simulink model "HVDCMMCInterconnection"  (R2023b)
settings: Solver=FixedStepDiscrete  StartTime=0.0  StopTime=10  FixedStep=Ts_Power  RelTol=1e-4
PreLoadFcn:
  | HVDCMMCInterconnectionParam
StartFcn:
  | tic
StopFcn:
  | toc
values from neighbouring files (symbols this model uses):
  C_PM = 1.758e-3    (= 0.001758)    [HVDCMMCInterconnectionParam.m]
  Cg = 50e-9    (= 5e-08)    [HVDCMMCInterconnectionParam.m]
  D_R = 0.001    [HVDCMMCInterconnectionParam.m]
  D_Rs = 1e8    (= 100000000)    [HVDCMMCInterconnectionParam.m]
  D_Vf = 0    [HVDCMMCInterconnectionParam.m]
  Fnom = 50    [HVDCMMCInterconnectionParam.m]
  HRM = 2    [HVDCMMCInterconnectionParam.m]
  Ki_Ireg = 6    [HVDCMMCInterconnectionParam.m]
  Ki_Preg = 1.0    (= 1)    [HVDCMMCInterconnectionParam.m]
  Ki_Qreg = 1.0    (= 1)    [HVDCMMCInterconnectionParam.m]
  Ki_VDCreg = 100    [HVDCMMCInterconnectionParam.m]
  Kp_Ireg = 0.6    [HVDCMMCInterconnectionParam.m]
  Kp_Preg = 0.5/3    (= 0.166666666667)    [HVDCMMCInterconnectionParam.m]
  Kp_Qreg = 0.5/3    (= 0.166666666667)    [HVDCMMCInterconnectionParam.m]
  Kp_VDCreg = 4    [HVDCMMCInterconnectionParam.m]
  L_cable = 15e-3    (= 0.015)    [HVDCMMCInterconnectionParam.m]
  Larm = Larm_pu*(Zb_ac/(2*pi*Fnom))    [HVDCMMCInterconnectionParam.m]
  Lff = Larm_pu/2    (= 0.075)    [HVDCMMCInterconnectionParam.m]
  Limits_Ireg = [ 2.0  -2.0]    [HVDCMMCInterconnectionParam.m]
  Limits_Preg = [ 1.2, 0.8 ]    [HVDCMMCInterconnectionParam.m]
  Limits_Qreg = [ 0.25, -0.25 ]    [HVDCMMCInterconnectionParam.m]
  Limits_VDCreg = [ 2.0  -2.0]    [HVDCMMCInterconnectionParam.m]
  Lxfo = 0.12    [HVDCMMCInterconnectionParam.m]
  Nb_PM = 36    [HVDCMMCInterconnectionParam.m]
  Pnom = 1000e6    (= 1000000000)    [HVDCMMCInterconnectionParam.m]
  R_cable = 0.5    [HVDCMMCInterconnectionParam.m]
  R_startup = 400    [HVDCMMCInterconnectionParam.m]
  Rarm = Rarm_pu*Zb_ac    [HVDCMMCInterconnectionParam.m]
  Rff = Rarm_pu/2    (= 0.00075)    [HVDCMMCInterconnectionParam.m]
  Rg = 100    [HVDCMMCInterconnectionParam.m]
  Rxfo = 0.003    [HVDCMMCInterconnectionParam.m]
  Slope_Pref = 0.5    [HVDCMMCInterconnectionParam.m]
  Slope_Qref = 0.5    [HVDCMMCInterconnectionParam.m]
  Slope_Vdc_ref = Vnom_dc/5    (= 128000)    [HVDCMMCInterconnectionParam.m]
  Tbrk1_On = 0.1    [HVDCMMCInterconnectionParam.m]
  Tbrk2_On = 1.0    (= 1)    [HVDCMMCInterconnectionParam.m]
  Tdeblock = 1.5    [HVDCMMCInterconnectionParam.m]
  Tfault = 9999    [HVDCMMCInterconnectionParam.m]
  Ton_Converter2 = 4    [HVDCMMCInterconnectionParam.m]
  Ton_PQreg = 4    [HVDCMMCInterconnectionParam.m]
  Ton_VDCreg = 1.5    [HVDCMMCInterconnectionParam.m]
  Ts = Ts_Control    (= 4e-05)    [HVDCMMCInterconnectionParam.m]    (also in power_circ2ss_sps_calc.m = 1e-06)
  Ts_Control = 40e-6    (= 4e-05)    [HVDCMMCInterconnectionParam.m]
  Ts_Power = 20e-6    (= 2e-05)    [HVDCMMCInterconnectionParam.m]
  Vb_ac = sqrt(2/3)*Vnom_sec    [HVDCMMCInterconnectionParam.m]
  Vb_dc = Vnom_dc    (= 640000)    [HVDCMMCInterconnectionParam.m]
  Vc0_PM = 0    [HVDCMMCInterconnectionParam.m]
  Vnom_dc = 640e3    (= 640000)    [HVDCMMCInterconnectionParam.m]
  Vnom_prim = 400e3    (= 400000)    [HVDCMMCInterconnectionParam.m]
  Vnom_sec = 333e3    (= 333000)    [HVDCMMCInterconnectionParam.m]
  w = 2*pi*Fnom    (= 314.159265359)    [HVDCMMCInterconnectionParam.m]
undefined symbols (not defined in the file or in its folder): ACDC, ACDC3, DiscIntNeverNeededParam, gcbh, Pcc, S, sps_AC, sps_rtmsupport
libraries: simulink x61, spsControlledVoltageSourceLib x56, spsCurrentMeasurementLib x56, spsDiodeLib x40, spsSeriesRLCBranchLib x32, spsVoltageMeasurementLib x20, powerlib_extras x9, spsHalfBridgeMMCmodel x8, spsGroundLib x7, spsSecondOrderFilterLib x6, spsabctodq0Lib x6, spsMeanLib x3
(part 8 of 11)

== system HVDCMMCInterconnection/MMC/An ==
  Uref : Inport
  Add1 : Sum  Commented=on  Inputs=+-
  Add2 : Sum  Commented=on  Inputs=-+
  An_Db : spsDiodeLib/Diode  Ron=D_R  Lon=0  Vf=D_Vf  IC=0  UseSnubber=0  Rs=D_Rs  Cs=D_Cs  Measurements=on
  An_Dt : spsDiodeLib/Diode  Ron=D_R  Lon=0  Vf=D_Vf  IC=0  UseSnubber=0  Rs=D_Rs  Cs=D_Cs  Measurements=on
  An_Icap : spsCurrentMeasurementLib/Current Measurement  PhasorSimulation=off  OutputType=Complex  PSBequivalent=0
  An_Ipos : spsCurrentMeasurementLib/Current Measurement  PhasorSimulation=off  OutputType=Complex  PSBequivalent=0
  An_Vbl : spsControlledVoltageSourceLib/Controlled Voltage Source  Initialize=on  Source_Type=AC  Amplitude=0  Phase=0  Frequency=0  Measurements=None
  An_Vin : spsControlledVoltageSourceLib/Controlled Voltage Source  Initialize=on  Source_Type=AC  Amplitude=0  Phase=0  Frequency=0  Measurements=None
  Bus Selector1 : BusSelector  OutputSignals=Diode current
  Bus Selector2 : BusSelector  OutputSignals=Diode current
  Compare To Constant1 : simulink/Logic and Bit Operations/Compare To Constant  Commented=on  relop=<=  const=0.5  OutDataTypeStr=boolean
  Constant3 : Constant  Commented=on  Value=ones(1,1)
  Constant4 : Constant  Commented=on  Value=ones(1,1)
  Data Type Conversion2 : DataTypeConversion  Commented=on  OutDataTypeStr=double  SaturateOnIntegerOverflow=off  RndMeth=Floor
  Demux : Demux  Outputs=2
  Demux2 : Demux  Outputs=2
  Demux5 : Demux  Outputs=2
  Discrete-Time Integrator1 : DiscreteIntegrator  IntegratorMethod=Integration: Trapezoidal  gainval=1  InitialCondition=Vc_Initial  SampleTime=Ts  UpperSaturationLimit=5000  LowerSaturationLimit=500  ICPrevOutput=DiscIntNeverNeededParam  ICPrevScaledInput=DiscIntNeverNeededParam
  From11 : From  Commented=on  GotoTag=uref
  From13 : From  Commented=on  GotoTag=Blk  TagVisibility=global
  Gain1 : Gain  Gain=n
  Gain4 : Gain  Gain=1/(C*n)
  Gain5 : Gain  Gain=2
  Mux1 : Mux  Inputs=2
  Mux2 : Mux  Inputs=2
  Mux3 : Mux  Commented=on  Inputs=2
  Mux7 : Mux  Inputs=2
  Product1 : Product  Commented=on
  Product3 : Product
  Product4 : Product
  Product5 : Product  Commented=on
  Product7 : Product
  Saturation : Saturate  Commented=on  UpperLimit=1  LowerLimit=-1
  Scope : Scope  Commented=on  NumInputPorts=2
  Sum3 : Sum  Inputs=1  InputSameDT=on  SaturateOnIntegerOverflow=on  OutDataTypeStr=Inherit: Same as first input
  Sum4 : Sum  Inputs=+-  InputSameDT=on  SaturateOnIntegerOverflow=on  OutDataTypeStr=Inherit: Same as first input
  Unit Delay5 : UnitDelay  InitialCondition=Vc_Initial  SampleTime=Ts  HasFrameUpgradeWarning=on
  Unit Delay6 : UnitDelay  InitialCondition=Vc_Initial  SampleTime=Ts  HasFrameUpgradeWarning=on
  Unit Delay7 : UnitDelay  SampleTime=Ts  HasFrameUpgradeWarning=on
  An_pos : PMIOPort  Side=Left
  An_neg : PMIOPort  Port=2  Side=Left
  Vc : Outport  VectorParamsAs1DForOutWhenUnconnected=off
  tag scope: An_Vbl_EMT=global, An_Vin_EMT=global, I_An_Db_EMT=global, I_An_Dt_EMT=global
  wires:
  Demux/1 -> [An_Vin_EMT]
  [An_Vin_EMT] -> An_Vin/1
  Product3/1 -> Sum3/1
  Demux/2 -> [An_Vbl_EMT]
  [Ipos] -> Mux1/1
  Unit Delay5/1 -> Sum4/2
  Gain5/1 -> Sum4/1
  Sum4/1 -> Product7/2, Product4/2, Vc/1  "Vc"
  Discrete-Time Integrator1/1 -> Unit Delay6/1
  Mux2/1 -> Demux/1
  [An_Vbl_EMT] -> An_Vbl/1
  [Icap] -> Mux1/2
  Gain4/1 -> Discrete-Time Integrator1/1
  Unit Delay6/1 -> Gain5/1, Unit Delay5/1
  Mux1/1 -> Unit Delay7/1
  Mux7/1 -> Gain1/1
  Demux2/1 -> Product4/1
  Demux2/2 -> Product7/1
  Product4/1 -> Mux2/1  "Vin"
  Product7/1 -> Mux2/2  "Vbl"
  Demux5/2 -> [ublk]
  [uref] -> Mux7/1
  [ublk] -> Mux7/2
  An_Ipos/1 -> [Ipos]
  An_Icap/1 -> [Icap]
  Unit Delay7/1 -> Product3/2
  Gain1/1 -> Demux2/1, Product3/1
  Demux5/1 -> [uref]
  Uref/1 -> Demux5/1
  Data Type Conversion2/1 -> Product5/1, Product1/1
  From13/1 -> Compare To Constant1/1
  Add2/1 -> Add1/2, Product5/2
  Constant4/1 -> Add1/1
  From11/1 -> Saturation/1
  Compare To Constant1/1 -> Data Type Conversion2/1
  Add1/1 -> Product1/2
  Product1/1 -> Mux3/1
  Constant3/1 -> Add2/2
  Saturation/1 -> Add2/1
  Sum3/1 -> Gain4/1
  Product5/1 -> Mux3/2
  Bus Selector2/1 -> [I_An_Dt_EMT]  "<Diode current>"
  An_Dt/1 -> Bus Selector2/1
  Bus Selector1/1 -> [I_An_Db_EMT]  "<Diode current>"
  An_Db/1 -> Bus Selector1/1
  connections:
  An_Ipos/RConn1 -- An_Dt/LConn1 -- An_Db/RConn1
  An_Vbl/LConn1 -- An_neg/RConn1 -- An_Db/LConn1
  An_Vbl/RConn1 -- An_Icap/RConn1
  An_Dt/RConn1 -- An_Icap/LConn1
  An_pos/RConn1 -- An_Vin/RConn1
  An_Vin/LConn1 -- An_Ipos/LConn1

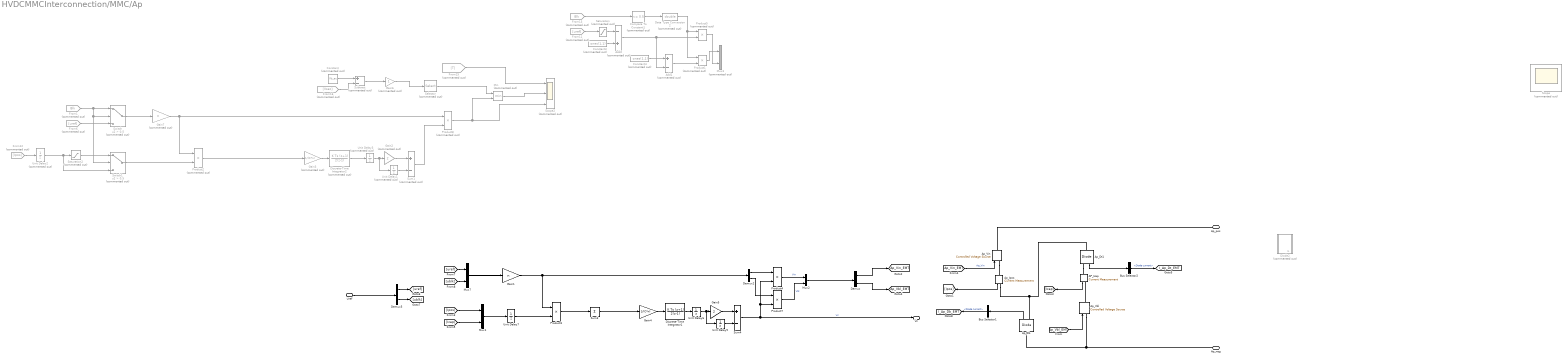
== system HVDCMMCInterconnection/MMC/Ap ==
  Uref : Inport
  AP_Icap : spsCurrentMeasurementLib/Current Measurement  PhasorSimulation=off  OutputType=Complex  PSBequivalent=0
  Add1 : Sum  Commented=on  Inputs=+-
  Add2 : Sum  Commented=on  Inputs=-+
  Ap_Db : spsDiodeLib/Diode  Ron=D_R  Lon=0  Vf=D_Vf  IC=0  UseSnubber=0  Rs=D_Rs  Cs=D_Cs  Measurements=on
  Ap_Dt1 : spsDiodeLib/Diode  Ron=D_R  Lon=0  Vf=D_Vf  IC=0  UseSnubber=0  Rs=D_Rs  Cs=D_Cs  Measurements=on
  Ap_Ipos : spsCurrentMeasurementLib/Current Measurement  PhasorSimulation=off  OutputType=Complex  PSBequivalent=0
  Ap_Vbl : spsControlledVoltageSourceLib/Controlled Voltage Source  Initialize=on  Source_Type=AC  Amplitude=0  Phase=0  Frequency=0  Measurements=None
  Ap_Vin : spsControlledVoltageSourceLib/Controlled Voltage Source  Initialize=on  Source_Type=AC  Amplitude=0  Phase=0  Frequency=0  Measurements=None
  Bus Selector1 : BusSelector  OutputSignals=Diode current
  Bus Selector2 : BusSelector  OutputSignals=Diode current
  Compare To Constant1 : simulink/Logic and Bit Operations/Compare To Constant  Commented=on  relop=<=  const=0.5  OutDataTypeStr=boolean
  Constant : Constant  Commented=on  Value=Vb_ac
  Constant3 : Constant  Commented=on  Value=ones(1,1)
  Constant4 : Constant  Commented=on  Value=ones(1,1)
  Data Type Conversion2 : DataTypeConversion  Commented=on  OutDataTypeStr=double  SaturateOnIntegerOverflow=off  RndMeth=Floor
  Demux : Demux  Outputs=2
  Demux2 : Demux  Outputs=2
  Demux5 : Demux  Outputs=2
  Diode2 : Subsystem  Commented=on  AncestorBlock=sps_lib/Power Electronics/Diode2  DialogController=POWERSYS.PowerSysDialog  LoadFcn=sps_rtmsupport('LoadFcn',gcbh);  StartFcn=sps_rtmsupport('StartFcn',gcbh);  StopFcn=sps_rtmsupport('StopFcn',gcbh);  mask(Diode){Ron=D_R, Lon=0, Vf=D_Vf, IC=0, UseSnubber=0, Rs=D_Rs, Cs=inf, Measurements=on}
      mask prompts: Ron "Resistance Ron (Ohms) :"; Lon "Inductance Lon (H) :"; Vf "Forward voltage Vf (V) :"; IC "Initial current Ic (A) :"; UseSnubber "Snubber"; Rs "Snubber resistance Rs (Ohms) :"; Cs "Snubber capacitance Cs (F) :"; Measurements "Show measurement port"
      mask help:
      | Implements a diode in parallel with a series RC snubber circuit.
      | In on-state the Diode model has an internal resistance (Ron) and inductance (Lon).
      | For most applications the internal inductance should be set to zero.
      | The Diode impedance is infinite in off-state mode.
      mask init:
      | block = gcb;
      | [WantBlockChoice,Ts,X,Y,Ron,Vf] = powericon('SwitchesInit','Diode',block,Rs,Cs,Ron,Vf);
      | powericon('SetInternalModels','set',block,WantBlockChoice);
      settings: LibrarySourceBlock=sps_lib/Power Electronics/Diode2  CopyFcn=sps_rtmsupport('CopyFcn',gcbh); powericon('SwitchesCopyFcn','Diode',gcb)  DeleteFcn=sps_rtmsupport('DeleteFcn',gcbh);  UndoDeleteFcn=sps_rtmsupport('UndoDeleteFcn',gcbh);  ModelCloseFcn=sps_rtmsupport('ModelCloseFcn',gcbh);  PreSaveFcn=sps_rtmsupport('PreSaveFcn',gcbh);  PostSaveFcn=sps_rtmsupport('PostSaveFcn',gcbh);  NameChangeFcn=sps_rtmsupport('NameChangeFcn',gcbh);  PreCopyFcn=sps_rtmsupport('PreCopyFcn',gcbh);  OpenFcn=sps_rtmsupport('OpenFcn',gcbh, [5 8]);  CloseFcn=sps_rtmsupport('CloseFcn',gcbh);  PreDeleteFcn=sps_rtmsupport('PreDeleteFcn',gcbh);
      mask Help: helpview(psbhelp);
      mask Callback Ron: powericon('SwitchesEnables',gcb,'Diode');
      mask Callback Measurements:
      | powericon('OutputMCback',gcb);
      | %sps_rtmsupport('parametereditingmodes',gcbh, [5 8]);
      mask Display: plot(X.p1,Y.p1,X.p2,Y.p2,X.p3,Y.p3,X.p4,Y.p4,X.p5,Y.p5,X.p6,Y.p6)
  Discrete-Time Integrator1 : DiscreteIntegrator  IntegratorMethod=Integration: Trapezoidal  gainval=1  InitialCondition=Vc_Initial  SampleTime=Ts  UpperSaturationLimit=5000  LowerSaturationLimit=500  ICPrevOutput=DiscIntNeverNeededParam  ICPrevScaledInput=DiscIntNeverNeededParam
  Discrete-Time Integrator2 : DiscreteIntegrator  Commented=on  IntegratorMethod=Integration: Trapezoidal  gainval=1  InitialCondition=Vc_Initial  SampleTime=Ts  UpperSaturationLimit=5000  LowerSaturationLimit=500  ICPrevOutput=DiscIntNeverNeededParam  ICPrevScaledInput=DiscIntNeverNeededParam
  From1 : From  Commented=on  GotoTag=Blk  TagVisibility=global
  From11 : From  Commented=on  GotoTag=uref
  From12 : From  Commented=on  GotoTag=Ipos
  From13 : From  Commented=on  GotoTag=Blk  TagVisibility=global
  From15 : From  Commented=on  GotoTag=T
  From16 : From  Commented=on  GotoTag=Vsec  TagVisibility=global
  From6 : From  Commented=on  GotoTag=uref
  Gain1 : Gain  Gain=n
  Gain2 : Gain  Commented=on  Gain=2
  Gain3 : Gain  Commented=on  Gain=1/(C*n)
  Gain4 : Gain  Gain=1/(C*n)
  Gain5 : Gain  Gain=2
  Gain6 : Gain  Commented=on
  Gain7 : Gain  Commented=on  Gain=n
  Min : MinMax  Commented=on  Inputs=2
  Mux1 : Mux  Inputs=2
  Mux2 : Mux  Inputs=2
  Mux3 : Mux  Commented=on  Inputs=2
  Mux7 : Mux  Inputs=2
  Product{1..2,5,8} (4 alike) : Product  Commented=on
  Product3 : Product
  Product4 : Product
  Product7 : Product
  Saturation : Saturate  Commented=on  UpperLimit=1  LowerLimit=-1
  Saturation2 : Saturate  Commented=on  UpperLimit=inf  LowerLimit=0
  Scope : Scope  Commented=on  NumInputPorts=2
  Scope2 : Scope  Commented=on  NumInputPorts=3
  Selector : Selector  Commented=on  InputPortWidth=3  IndexOptions=Index vector (dialog)  Indices=[1]  OutputSizes=1
  Subtract : Sum  Commented=on  Inputs=+-
  Sum1 : Sum  Commented=on  Inputs=+-  InputSameDT=on  SaturateOnIntegerOverflow=on  OutDataTypeStr=Inherit: Same as first input
  Sum3 : Sum  Inputs=1  InputSameDT=on  SaturateOnIntegerOverflow=on  OutDataTypeStr=Inherit: Same as first input
  Sum4 : Sum  Inputs=+-  InputSameDT=on  SaturateOnIntegerOverflow=on  OutDataTypeStr=Inherit: Same as first input
  Switch : Switch  Commented=on  Criteria=u2 > Threshold  Threshold=0.5  SaturateOnIntegerOverflow=off  InputSameDT=off
  Switch1 : Switch  Commented=on  Criteria=u2 > Threshold  Threshold=0.5  SaturateOnIntegerOverflow=off  InputSameDT=off
  Unit Delay1 : UnitDelay  Commented=on  InitialCondition=Vc_Initial  SampleTime=Ts  HasFrameUpgradeWarning=on
  Unit Delay2 : UnitDelay  Commented=on  SampleTime=Ts  HasFrameUpgradeWarning=on
  Unit Delay3 : UnitDelay  Commented=on  InitialCondition=Vc_Initial  SampleTime=Ts  HasFrameUpgradeWarning=on
  Unit Delay5 : UnitDelay  InitialCondition=Vc_Initial  SampleTime=Ts  HasFrameUpgradeWarning=on
  Unit Delay6 : UnitDelay  InitialCondition=Vc_Initial  SampleTime=Ts  HasFrameUpgradeWarning=on
  Unit Delay7 : UnitDelay  SampleTime=Ts  HasFrameUpgradeWarning=on
  Ap_pos : PMIOPort  Side=Left
  Ap_neg : PMIOPort  Port=2  Side=Left
  Vc : Outport  VectorParamsAs1DForOutWhenUnconnected=off
  tag scope: Ap_Vbl_EMT=global, Ap_Vin_EMT=global, I_Ap_Db_EMT=global, I_Ap_Dt_EMT=global
  wires:
  Demux/1 -> [Ap_Vin_EMT]
  [Ap_Vin_EMT] -> Ap_Vin/1  "Ap_Vin"
  Product3/1 -> Sum3/1
  Demux/2 -> [Ap_Vbl_EMT]
  [Ipos] -> Mux1/1
  Unit Delay5/1 -> Sum4/2
  Gain5/1 -> Sum4/1
  Sum4/1 -> Product7/2, Product4/2, Vc/1  "Vc"
  Discrete-Time Integrator1/1 -> Unit Delay6/1
  Mux2/1 -> Demux/1
  [Ap_Vbl_EMT] -> Ap_Vbl/1
  [Icap] -> Mux1/2
  Gain4/1 -> Discrete-Time Integrator1/1
  Unit Delay6/1 -> Gain5/1, Unit Delay5/1
  Mux1/1 -> Unit Delay7/1
  Mux7/1 -> Gain1/1
  Demux2/1 -> Product4/1
  Demux2/2 -> Product7/1
  Product4/1 -> Mux2/1  "Vin"
  Product7/1 -> Mux2/2  "Vbl"
  Demux5/2 -> [ublk]
  [uref] -> Mux7/1
  [ublk] -> Mux7/2
  Ap_Ipos/1 -> [Ipos]
  AP_Icap/1 -> [Icap]
  Unit Delay7/1 -> Product3/2
  Gain1/1 -> Demux2/1, Product3/1
  Demux5/1 -> [uref]
  Uref/1 -> Demux5/1
  Data Type Conversion2/1 -> Product5/1, Product1/1
  From13/1 -> Compare To Constant1/1
  Add2/1 -> Add1/2, Product5/2
  Constant4/1 -> Add1/1
  From11/1 -> Saturation/1
  Compare To Constant1/1 -> Data Type Conversion2/1
  Add1/1 -> Product1/2
  Product1/1 -> Mux3/1
  Constant3/1 -> Add2/2
  Saturation/1 -> Add2/1
  Sum3/1 -> Gain4/1
  Product5/1 -> Mux3/2
  From1/1 -> Switch1/2, Switch/2, Switch/1
  Saturation2/1 -> Switch1/1
  Gain7/1 -> Product2/1, Product8/1
  Unit Delay3/1 -> Gain2/1, Unit Delay1/1
  Sum1/1 -> Product8/2
  Switch/1 -> Gain7/1
  Switch1/1 -> Product2/2
  From6/1 -> Switch/3
  Unit Delay2/1 -> Saturation2/1, Switch1/3
  Gain3/1 -> Discrete-Time Integrator2/1
  Discrete-Time Integrator2/1 -> Unit Delay3/1
  Unit Delay1/1 -> Sum1/2
  From12/1 -> Unit Delay2/1
  Product2/1 -> Gain3/1
  Gain2/1 -> Sum1/1
  Product8/1 -> Min/2, Scope2/3
  From16/1 -> Subtract/2
  Constant/1 -> Subtract/1
  Subtract/1 -> Gain6/1
  Gain6/1 -> Selector/1
  Selector/1 -> Min/1
  Min/1 -> Scope2/2
  From15/1 -> Scope2/1
  Bus Selector1/1 -> [I_Ap_Db_EMT]  "<Diode current>"
  Ap_Db/1 -> Bus Selector1/1
  Ap_Dt1/1 -> Bus Selector2/1
  Bus Selector2/1 -> [I_Ap_Dt_EMT]  "<Diode current>"
  connections:
  Ap_Ipos/RConn1 -- Ap_Dt1/LConn1 -- Ap_Db/RConn1
  Ap_Vbl/LConn1 -- Ap_neg/RConn1 -- Ap_Db/LConn1
  Ap_Vbl/RConn1 -- AP_Icap/RConn1
  Ap_Dt1/RConn1 -- AP_Icap/LConn1
  Ap_pos/RConn1 -- Ap_Vin/RConn1
  Ap_Vin/LConn1 -- Ap_Ipos/LConn1

== system HVDCMMCInterconnection/MMC/Bn ==
  Uref : Inport
  Bn_Db : spsDiodeLib/Diode  Ron=D_R  Lon=0  Vf=D_Vf  IC=0  UseSnubber=0  Rs=D_Rs  Cs=D_Cs  Measurements=on
  Bn_Dt : spsDiodeLib/Diode  Ron=D_R  Lon=0  Vf=D_Vf  IC=0  UseSnubber=0  Rs=D_Rs  Cs=D_Cs  Measurements=on
  Bn_Icap : spsCurrentMeasurementLib/Current Measurement  PhasorSimulation=off  OutputType=Complex  PSBequivalent=0
  Bn_Ipos : spsCurrentMeasurementLib/Current Measurement  PhasorSimulation=off  OutputType=Complex  PSBequivalent=0
  Bn_Vbl : spsControlledVoltageSourceLib/Controlled Voltage Source  Initialize=on  Source_Type=AC  Amplitude=0  Phase=0  Frequency=0  Measurements=None
  Bn_Vin : spsControlledVoltageSourceLib/Controlled Voltage Source  Initialize=on  Source_Type=AC  Amplitude=0  Phase=0  Frequency=0  Measurements=None
  Bus Selector1 : BusSelector  OutputSignals=Diode current
  Bus Selector2 : BusSelector  OutputSignals=Diode current
  Demux : Demux  Outputs=2
  Demux2 : Demux  Outputs=2
  Demux5 : Demux  Outputs=2
  Discrete-Time Integrator1 : DiscreteIntegrator  IntegratorMethod=Integration: Trapezoidal  gainval=1  InitialCondition=Vc_Initial  SampleTime=Ts  UpperSaturationLimit=5000  LowerSaturationLimit=500  ICPrevOutput=DiscIntNeverNeededParam  ICPrevScaledInput=DiscIntNeverNeededParam
  Gain1 : Gain  Gain=n
  Gain4 : Gain  Gain=1/(C*n)
  Gain5 : Gain  Gain=2
  Mux1 : Mux  Inputs=2
  Mux2 : Mux  Inputs=2
  Mux7 : Mux  Inputs=2
  Product3 : Product
  Product4 : Product
  Product7 : Product
  Sum3 : Sum  Inputs=1  InputSameDT=on  SaturateOnIntegerOverflow=on  OutDataTypeStr=Inherit: Same as first input
  Sum4 : Sum  Inputs=+-  InputSameDT=on  SaturateOnIntegerOverflow=on  OutDataTypeStr=Inherit: Same as first input
  Unit Delay5 : UnitDelay  InitialCondition=Vc_Initial  SampleTime=Ts  HasFrameUpgradeWarning=on
  Unit Delay6 : UnitDelay  InitialCondition=Vc_Initial  SampleTime=Ts  HasFrameUpgradeWarning=on
  Unit Delay7 : UnitDelay  SampleTime=Ts  HasFrameUpgradeWarning=on
  Bn_pos : PMIOPort  Side=Left
  Bn_neg : PMIOPort  Port=2  Side=Left
  Vc : Outport  VectorParamsAs1DForOutWhenUnconnected=off
  tag scope: Bn_Vbl_EMT=global, Bn_Vin_EMT=global, I_Bn_Db_EMT=global, I_Bn_Dt_EMT=global
  wires:
  Demux/1 -> [Bn_Vin_EMT]
  [Bn_Vin_EMT] -> Bn_Vin/1
  Product3/1 -> Sum3/1
  Demux/2 -> [Bn_Vbl_EMT]
  [Ipos] -> Mux1/1
  Unit Delay5/1 -> Sum4/2
  Gain5/1 -> Sum4/1
  Sum4/1 -> Product7/2, Product4/2, Vc/1  "Vc"
  Discrete-Time Integrator1/1 -> Unit Delay6/1
  Mux2/1 -> Demux/1
  [Bn_Vbl_EMT] -> Bn_Vbl/1
  [Icap] -> Mux1/2
  Gain4/1 -> Discrete-Time Integrator1/1
  Unit Delay6/1 -> Gain5/1, Unit Delay5/1
  Mux1/1 -> Unit Delay7/1
  Mux7/1 -> Gain1/1
  Demux2/1 -> Product4/1
  Demux2/2 -> Product7/1
  Product4/1 -> Mux2/1  "Vin"
  Product7/1 -> Mux2/2  "Vbl"
  Demux5/2 -> [ublk]
  [uref] -> Mux7/1
  [ublk] -> Mux7/2
  Bn_Ipos/1 -> [Ipos]
  Bn_Icap/1 -> [Icap]
  Unit Delay7/1 -> Product3/2
  Gain1/1 -> Demux2/1, Product3/1
  Demux5/1 -> [uref]
  Uref/1 -> Demux5/1
  Sum3/1 -> Gain4/1
  Bus Selector2/1 -> [I_Bn_Dt_EMT]  "<Diode current>"
  Bn_Dt/1 -> Bus Selector2/1
  Bus Selector1/1 -> [I_Bn_Db_EMT]  "<Diode current>"
  Bn_Db/1 -> Bus Selector1/1
  connections:
  Bn_Ipos/RConn1 -- Bn_Dt/LConn1 -- Bn_Db/RConn1
  Bn_Vbl/LConn1 -- Bn_neg/RConn1 -- Bn_Db/LConn1
  Bn_Vbl/RConn1 -- Bn_Icap/RConn1
  Bn_Dt/RConn1 -- Bn_Icap/LConn1
  Bn_pos/RConn1 -- Bn_Vin/RConn1
  Bn_Vin/LConn1 -- Bn_Ipos/LConn1

== system HVDCMMCInterconnection/MMC/Bp ==
  Uref : Inport
  BP_Icap : spsCurrentMeasurementLib/Current Measurement  PhasorSimulation=off  OutputType=Complex  PSBequivalent=0
  Bp_Db : spsDiodeLib/Diode  Ron=D_R  Lon=0  Vf=D_Vf  IC=0  UseSnubber=0  Rs=D_Rs  Cs=D_Cs  Measurements=on
  Bp_Dt : spsDiodeLib/Diode  Ron=D_R  Lon=0  Vf=D_Vf  IC=0  UseSnubber=0  Rs=D_Rs  Cs=D_Cs  Measurements=on
  Bp_Ipos : spsCurrentMeasurementLib/Current Measurement  PhasorSimulation=off  OutputType=Complex  PSBequivalent=0
  Bp_Vbl : spsControlledVoltageSourceLib/Controlled Voltage Source  Initialize=on  Source_Type=AC  Amplitude=0  Phase=0  Frequency=0  Measurements=None
  Bp_Vin : spsControlledVoltageSourceLib/Controlled Voltage Source  Initialize=on  Source_Type=AC  Amplitude=0  Phase=0  Frequency=0  Measurements=None
  Bus Selector1 : BusSelector  OutputSignals=Diode current
  Bus Selector2 : BusSelector  OutputSignals=Diode current
  Demux : Demux  Outputs=2
  Demux2 : Demux  Outputs=2
  Demux5 : Demux  Outputs=2
  Discrete-Time Integrator1 : DiscreteIntegrator  IntegratorMethod=Integration: Trapezoidal  gainval=1  InitialCondition=Vc_Initial  SampleTime=Ts  UpperSaturationLimit=5000  LowerSaturationLimit=500  ICPrevOutput=DiscIntNeverNeededParam  ICPrevScaledInput=DiscIntNeverNeededParam
  Gain1 : Gain  Gain=n
  Gain4 : Gain  Gain=1/(C*n)
  Gain5 : Gain  Gain=2
  Mux1 : Mux  Inputs=2
  Mux2 : Mux  Inputs=2
  Mux7 : Mux  Inputs=2
  Product3 : Product
  Product4 : Product
  Product7 : Product
  Sum3 : Sum  Inputs=1  InputSameDT=on  SaturateOnIntegerOverflow=on  OutDataTypeStr=Inherit: Same as first input
  Sum4 : Sum  Inputs=+-  InputSameDT=on  SaturateOnIntegerOverflow=on  OutDataTypeStr=Inherit: Same as first input
  Unit Delay5 : UnitDelay  InitialCondition=Vc_Initial  SampleTime=Ts  HasFrameUpgradeWarning=on
  Unit Delay6 : UnitDelay  InitialCondition=Vc_Initial  SampleTime=Ts  HasFrameUpgradeWarning=on
  Unit Delay7 : UnitDelay  SampleTime=Ts  HasFrameUpgradeWarning=on
  Bp_pos : PMIOPort  Side=Left
  Bp_neg : PMIOPort  Port=2  Side=Left
  Vc : Outport  VectorParamsAs1DForOutWhenUnconnected=off
  tag scope: Bp_Vbl_EMT=global, Bp_Vin_EMT=global, I_Bp_Db_EMT=global, I_Bp_Dt_EMT=global
  wires:
  Demux/1 -> [Bp_Vin_EMT]
  [Bp_Vin_EMT] -> Bp_Vin/1
  Product3/1 -> Sum3/1
  Demux/2 -> [Bp_Vbl_EMT]
  [Ipos] -> Mux1/1
  Unit Delay5/1 -> Sum4/2
  Gain5/1 -> Sum4/1
  Sum4/1 -> Product7/2, Product4/2, Vc/1  "Vc"
  Discrete-Time Integrator1/1 -> Unit Delay6/1
  Mux2/1 -> Demux/1
  [Bp_Vbl_EMT] -> Bp_Vbl/1
  [Icap] -> Mux1/2
  Gain4/1 -> Discrete-Time Integrator1/1
  Unit Delay6/1 -> Gain5/1, Unit Delay5/1
  Mux1/1 -> Unit Delay7/1
  Mux7/1 -> Gain1/1
  Demux2/1 -> Product4/1
  Demux2/2 -> Product7/1
  Product4/1 -> Mux2/1  "Vin"
  Product7/1 -> Mux2/2  "Vbl"
  Demux5/2 -> [ublk]
  [uref] -> Mux7/1
  [ublk] -> Mux7/2
  Bp_Ipos/1 -> [Ipos]
  BP_Icap/1 -> [Icap]
  Unit Delay7/1 -> Product3/2
  Gain1/1 -> Demux2/1, Product3/1
  Demux5/1 -> [uref]
  Uref/1 -> Demux5/1
  Sum3/1 -> Gain4/1
  Bus Selector2/1 -> [I_Bp_Dt_EMT]  "<Diode current>"
  Bp_Db/1 -> Bus Selector1/1
  Bus Selector1/1 -> [I_Bp_Db_EMT]  "<Diode current>"
  Bp_Dt/1 -> Bus Selector2/1
  connections:
  Bp_Ipos/RConn1 -- Bp_Dt/LConn1 -- Bp_Db/RConn1
  Bp_Vbl/LConn1 -- Bp_neg/RConn1 -- Bp_Db/LConn1
  Bp_Vbl/RConn1 -- BP_Icap/RConn1
  Bp_Dt/RConn1 -- BP_Icap/LConn1
  Bp_pos/RConn1 -- Bp_Vin/RConn1
  Bp_Vin/LConn1 -- Bp_Ipos/LConn1

== system HVDCMMCInterconnection/MMC/Cn ==
  Uref : Inport
  Bus Selector1 : BusSelector  OutputSignals=Diode current
  Bus Selector2 : BusSelector  OutputSignals=Diode current
  Cn_Db : spsDiodeLib/Diode  Ron=D_R  Lon=0  Vf=D_Vf  IC=0  UseSnubber=0  Rs=D_Rs  Cs=D_Cs  Measurements=on
  Cn_Dt : spsDiodeLib/Diode  Ron=D_R  Lon=0  Vf=D_Vf  IC=0  UseSnubber=0  Rs=D_Rs  Cs=D_Cs  Measurements=on
  Cn_Icap : spsCurrentMeasurementLib/Current Measurement  PhasorSimulation=off  OutputType=Complex  PSBequivalent=0
  Cn_Ipos : spsCurrentMeasurementLib/Current Measurement  PhasorSimulation=off  OutputType=Complex  PSBequivalent=0
  Cn_Vbl : spsControlledVoltageSourceLib/Controlled Voltage Source  Initialize=on  Source_Type=AC  Amplitude=0  Phase=0  Frequency=0  Measurements=None
  Cn_Vin : spsControlledVoltageSourceLib/Controlled Voltage Source  Initialize=on  Source_Type=AC  Amplitude=0  Phase=0  Frequency=0  Measurements=None
  Demux : Demux  Outputs=2
  Demux2 : Demux  Outputs=2
  Demux5 : Demux  Outputs=2
  Discrete-Time Integrator1 : DiscreteIntegrator  IntegratorMethod=Integration: Trapezoidal  gainval=1  InitialCondition=Vc_Initial  SampleTime=Ts  UpperSaturationLimit=5000  LowerSaturationLimit=500  ICPrevOutput=DiscIntNeverNeededParam  ICPrevScaledInput=DiscIntNeverNeededParam
  Gain1 : Gain  Gain=n
  Gain4 : Gain  Gain=1/(C*n)
  Gain5 : Gain  Gain=2
  Mux1 : Mux  Inputs=2
  Mux2 : Mux  Inputs=2
  Mux7 : Mux  Inputs=2
  Product3 : Product
  Product4 : Product
  Product7 : Product
  Sum3 : Sum  Inputs=1  InputSameDT=on  SaturateOnIntegerOverflow=on  OutDataTypeStr=Inherit: Same as first input
  Sum4 : Sum  Inputs=+-  InputSameDT=on  SaturateOnIntegerOverflow=on  OutDataTypeStr=Inherit: Same as first input
  Unit Delay5 : UnitDelay  InitialCondition=Vc_Initial  SampleTime=Ts  HasFrameUpgradeWarning=on
  Unit Delay6 : UnitDelay  InitialCondition=Vc_Initial  SampleTime=Ts  HasFrameUpgradeWarning=on
  Unit Delay7 : UnitDelay  SampleTime=Ts  HasFrameUpgradeWarning=on
  Cn_pos : PMIOPort  Side=Left
  Cn_neg : PMIOPort  Port=2  Side=Left
  Vc : Outport  VectorParamsAs1DForOutWhenUnconnected=off
  tag scope: Cn_Vbl_EMT=global, Cn_Vin_EMT=global, I_Cn_Db_EMT=global, I_Cn_Dt_EMT=global
  wires:
  Demux/1 -> [Cn_Vin_EMT]
  [Cn_Vin_EMT] -> Cn_Vin/1
  Product3/1 -> Sum3/1
  Demux/2 -> [Cn_Vbl_EMT]
  [Ipos] -> Mux1/1
  Unit Delay5/1 -> Sum4/2
  Gain5/1 -> Sum4/1
  Sum4/1 -> Product7/2, Product4/2, Vc/1  "Vc"
  Discrete-Time Integrator1/1 -> Unit Delay6/1
  Mux2/1 -> Demux/1
  [Cn_Vbl_EMT] -> Cn_Vbl/1
  [Icap] -> Mux1/2
  Gain4/1 -> Discrete-Time Integrator1/1
  Unit Delay6/1 -> Gain5/1, Unit Delay5/1
  Mux1/1 -> Unit Delay7/1
  Mux7/1 -> Gain1/1
  Demux2/1 -> Product4/1
  Demux2/2 -> Product7/1
  Product4/1 -> Mux2/1  "Vin"
  Product7/1 -> Mux2/2  "Vbl"
  Demux5/2 -> [ublk]
  [uref] -> Mux7/1
  [ublk] -> Mux7/2
  Cn_Ipos/1 -> [Ipos]
  Cn_Icap/1 -> [Icap]
  Unit Delay7/1 -> Product3/2
  Gain1/1 -> Demux2/1, Product3/1
  Demux5/1 -> [uref]
  Uref/1 -> Demux5/1
  Sum3/1 -> Gain4/1
  Bus Selector1/1 -> [I_Cn_Db_EMT]  "<Diode current>"
  Bus Selector2/1 -> [I_Cn_Dt_EMT]  "<Diode current>"
  Cn_Dt/1 -> Bus Selector2/1
  Cn_Db/1 -> Bus Selector1/1
  connections:
  Cn_Ipos/RConn1 -- Cn_Dt/LConn1 -- Cn_Db/RConn1
  Cn_Vbl/LConn1 -- Cn_neg/RConn1 -- Cn_Db/LConn1
  Cn_Vbl/RConn1 -- Cn_Icap/RConn1
  Cn_Dt/RConn1 -- Cn_Icap/LConn1
  Cn_pos/RConn1 -- Cn_Vin/RConn1
  Cn_Vin/LConn1 -- Cn_Ipos/LConn1

== system HVDCMMCInterconnection/MMC/Cp ==
  Uref : Inport
  Bus Selector1 : BusSelector  OutputSignals=Diode current
  Bus Selector2 : BusSelector  OutputSignals=Diode current
  CP_Icap : spsCurrentMeasurementLib/Current Measurement  PhasorSimulation=off  OutputType=Complex  PSBequivalent=0
  Cp_Db : spsDiodeLib/Diode  Ron=D_R  Lon=0  Vf=D_Vf  IC=0  UseSnubber=0  Rs=D_Rs  Cs=D_Cs  Measurements=on
  Cp_Dt : spsDiodeLib/Diode  Ron=D_R  Lon=0  Vf=D_Vf  IC=0  UseSnubber=0  Rs=D_Rs  Cs=D_Cs  Measurements=on
  Cp_Ipos : spsCurrentMeasurementLib/Current Measurement  PhasorSimulation=off  OutputType=Complex  PSBequivalent=0
  Cp_Vbl : spsControlledVoltageSourceLib/Controlled Voltage Source  Initialize=on  Source_Type=AC  Amplitude=0  Phase=0  Frequency=0  Measurements=None
  Cp_Vin : spsControlledVoltageSourceLib/Controlled Voltage Source  Initialize=on  Source_Type=AC  Amplitude=0  Phase=0  Frequency=0  Measurements=None
  Demux : Demux  Outputs=2
  Demux2 : Demux  Outputs=2
  Demux5 : Demux  Outputs=2
  Discrete-Time Integrator1 : DiscreteIntegrator  IntegratorMethod=Integration: Trapezoidal  gainval=1  InitialCondition=Vc_Initial  SampleTime=Ts  UpperSaturationLimit=5000  LowerSaturationLimit=500  ICPrevOutput=DiscIntNeverNeededParam  ICPrevScaledInput=DiscIntNeverNeededParam
  Gain1 : Gain  Gain=n
  Gain4 : Gain  Gain=1/(C*n)
  Gain5 : Gain  Gain=2
  Mux1 : Mux  Inputs=2
  Mux2 : Mux  Inputs=2
  Mux7 : Mux  Inputs=2
  Product3 : Product
  Product4 : Product
  Product7 : Product
  Sum3 : Sum  Inputs=1  InputSameDT=on  SaturateOnIntegerOverflow=on  OutDataTypeStr=Inherit: Same as first input
  Sum4 : Sum  Inputs=+-  InputSameDT=on  SaturateOnIntegerOverflow=on  OutDataTypeStr=Inherit: Same as first input
  Unit Delay5 : UnitDelay  InitialCondition=Vc_Initial  SampleTime=Ts  HasFrameUpgradeWarning=on
  Unit Delay6 : UnitDelay  InitialCondition=Vc_Initial  SampleTime=Ts  HasFrameUpgradeWarning=on
  Unit Delay7 : UnitDelay  SampleTime=Ts  HasFrameUpgradeWarning=on
  Cp_pos : PMIOPort  Side=Left
  Cp_neg : PMIOPort  Port=2  Side=Left
  Vc : Outport  VectorParamsAs1DForOutWhenUnconnected=off
  tag scope: Cp_Vbl_EMT=global, Cp_Vin_EMT=global, I_Cp_Db_EMT=global, I_Cp_Dt_EMT=global
  wires:
  Demux/1 -> [Cp_Vin_EMT]
  [Cp_Vin_EMT] -> Cp_Vin/1
  Product3/1 -> Sum3/1
  Demux/2 -> [Cp_Vbl_EMT]
  [Ipos] -> Mux1/1
  Unit Delay5/1 -> Sum4/2
  Gain5/1 -> Sum4/1
  Sum4/1 -> Product7/2, Product4/2, Vc/1  "Vc"
  Discrete-Time Integrator1/1 -> Unit Delay6/1
  Mux2/1 -> Demux/1
  [Cp_Vbl_EMT] -> Cp_Vbl/1
  [Icap] -> Mux1/2
  Gain4/1 -> Discrete-Time Integrator1/1
  Unit Delay6/1 -> Gain5/1, Unit Delay5/1
  Mux1/1 -> Unit Delay7/1
  Mux7/1 -> Gain1/1
  Demux2/1 -> Product4/1
  Demux2/2 -> Product7/1
  Product4/1 -> Mux2/1  "Vin"
  Product7/1 -> Mux2/2  "Vbl"
  Demux5/2 -> [ublk]
  [uref] -> Mux7/1
  [ublk] -> Mux7/2
  Cp_Ipos/1 -> [Ipos]
  CP_Icap/1 -> [Icap]
  Unit Delay7/1 -> Product3/2
  Gain1/1 -> Demux2/1, Product3/1
  Demux5/1 -> [uref]
  Uref/1 -> Demux5/1
  Sum3/1 -> Gain4/1
  Bus Selector2/1 -> [I_Cp_Dt_EMT]  "<Diode current>"
  Cp_Db/1 -> Bus Selector1/1
  Bus Selector1/1 -> [I_Cp_Db_EMT]  "<Diode current>"
  Cp_Dt/1 -> Bus Selector2/1
  connections:
  Cp_Ipos/RConn1 -- Cp_Dt/LConn1 -- Cp_Db/RConn1
  Cp_Vbl/LConn1 -- Cp_neg/RConn1 -- Cp_Db/LConn1
  Cp_Vbl/RConn1 -- CP_Icap/RConn1
  Cp_Dt/RConn1 -- CP_Icap/LConn1
  Cp_pos/RConn1 -- Cp_Vin/RConn1
  Cp_Vin/LConn1 -- Cp_Ipos/LConn1

== system HVDCMMCInterconnection/MMC/Half-Bridge MMC Ap (Aggregate model of 36 PM)2 ==
  Uref : Inport
  Controlled Voltage Source : spsControlledVoltageSourceLib/Controlled Voltage Source  Initialize=on  Source_Type=AC  Amplitude=0  Phase=0  Frequency=0  Measurements=None
  Controlled Voltage Source1 : spsControlledVoltageSourceLib/Controlled Voltage Source  Initialize=on  Source_Type=AC  Amplitude=0  Phase=0  Frequency=0  Measurements=None
  Current Measurement : spsCurrentMeasurementLib/Current Measurement  PhasorSimulation=off  OutputType=Complex  PSBequivalent=0
  Current Measurement1 : spsCurrentMeasurementLib/Current Measurement  PhasorSimulation=off  OutputType=Complex  PSBequivalent=0
  Demux : Demux  Outputs=2
  Diode : spsDiodeLib/Diode  Ron=Ron_Diode  Lon=0  Vf=Vf_Diode  IC=0  UseSnubber=0  Rs=Rs_Diode  Cs=Cs_Diode  Measurements=off
  Diode1 : spsDiodeLib/Diode  Ron=Ron_Diode  Lon=0  Vf=Vf_Diode  IC=0  UseSnubber=0  Rs=Rs_Diode  Cs=Cs_Diode  Measurements=off
  Discrete-Time Integrator1 : DiscreteIntegrator  IntegratorMethod=Integration: Trapezoidal  gainval=1  InitialCondition=Vc_Initial  SampleTime=Ts  UpperSaturationLimit=5000  LowerSaturationLimit=500  ICPrevOutput=DiscIntNeverNeededParam  ICPrevScaledInput=DiscIntNeverNeededParam
  Gain1 : Gain  Gain=n
  Gain4 : Gain  Gain=1/(C*n)
  Gain5 : Gain  Gain=2
  Mux1 : Mux  Inputs=2
  Product3 : Product
  Product4 : Product
  Sum3 : Sum  Inputs=1  InputSameDT=on  SaturateOnIntegerOverflow=on  OutDataTypeStr=Inherit: Same as first input
  Sum4 : Sum  Inputs=+-  InputSameDT=on  SaturateOnIntegerOverflow=on  OutDataTypeStr=Inherit: Same as first input
  Unit Delay2 : UnitDelay  SampleTime=Ts  HasFrameUpgradeWarning=on
  Unit Delay5 : UnitDelay  InitialCondition=Vc_Initial  SampleTime=Ts  HasFrameUpgradeWarning=on
  Unit Delay6 : UnitDelay  InitialCondition=Vc_Initial  SampleTime=Ts  HasFrameUpgradeWarning=on
  1 : PMIOPort  Side=Left
  2 : PMIOPort  Port=2  Side=Left
  Vc : Outport  VectorParamsAs1DForOutWhenUnconnected=off
  wires:
  Demux/1 -> [Vin]
  [Vin] -> Controlled Voltage Source/1
  Current Measurement1/1 -> [Icap]
  Product3/1 -> Sum3/1
  Demux/2 -> [Vbl]
  [Imod] -> Mux1/1
  Sum3/1 -> Gain4/1
  Unit Delay5/1 -> Sum4/2
  Gain5/1 -> Sum4/1
  Mux1/1 -> Unit Delay2/1
  Uref/1 -> Gain1/1
  Sum4/1 -> Vc/1, Product4/2
  Current Measurement/1 -> [Imod]
  Unit Delay2/1 -> Product3/2
  Discrete-Time Integrator1/1 -> Unit Delay6/1
  Product4/1 -> Demux/1
  [Vbl] -> Controlled Voltage Source1/1
  [Icap] -> Mux1/2
  Gain4/1 -> Discrete-Time Integrator1/1
  Unit Delay6/1 -> Gain5/1, Unit Delay5/1
  Gain1/1 -> Product3/1, Product4/1
  connections:
  Diode1/LConn1 -- Current Measurement/RConn1 -- Diode/RConn1
  Controlled Voltage Source1/LConn1 -- Diode/LConn1 -- 2/RConn1
  Controlled Voltage Source1/RConn1 -- Current Measurement1/RConn1
  Diode1/RConn1 -- Current Measurement1/LConn1
  1/RConn1 -- Controlled Voltage Source/RConn1
  Controlled Voltage Source/LConn1 -- Current Measurement/LConn1

== system HVDCMMCInterconnection/MMC/Half-Bridge MMC Ap (Aggregate model of 36 PM)7 ==
  Uref : Inport
  Controlled Voltage Source : spsControlledVoltageSourceLib/Controlled Voltage Source  Initialize=on  Source_Type=AC  Amplitude=0  Phase=0  Frequency=0  Measurements=None
  Controlled Voltage Source1 : spsControlledVoltageSourceLib/Controlled Voltage Source  Initialize=on  Source_Type=AC  Amplitude=0  Phase=0  Frequency=0  Measurements=None
  Current Measurement : spsCurrentMeasurementLib/Current Measurement  PhasorSimulation=off  OutputType=Complex  PSBequivalent=0
  Current Measurement1 : spsCurrentMeasurementLib/Current Measurement  PhasorSimulation=off  OutputType=Complex  PSBequivalent=0
  Demux : Demux  Outputs=2
  Diode : spsDiodeLib/Diode  Ron=Ron_Diode  Lon=0  Vf=Vf_Diode  IC=0  UseSnubber=0  Rs=Rs_Diode  Cs=Cs_Diode  Measurements=off
  Diode1 : spsDiodeLib/Diode  Ron=Ron_Diode  Lon=0  Vf=Vf_Diode  IC=0  UseSnubber=0  Rs=Rs_Diode  Cs=Cs_Diode  Measurements=off
  Discrete-Time Integrator1 : DiscreteIntegrator  IntegratorMethod=Integration: Trapezoidal  gainval=1  InitialCondition=Vc_Initial  SampleTime=Ts  UpperSaturationLimit=5000  LowerSaturationLimit=500  ICPrevOutput=DiscIntNeverNeededParam  ICPrevScaledInput=DiscIntNeverNeededParam
  Gain1 : Gain  Gain=n
  Gain4 : Gain  Gain=1/(C*n)
  Gain5 : Gain  Gain=2
  Mux1 : Mux  Inputs=2
  Product3 : Product
  Product4 : Product
  Scope : Scope  NumInputPorts=3
  Sum3 : Sum  Inputs=1  InputSameDT=on  SaturateOnIntegerOverflow=on  OutDataTypeStr=Inherit: Same as first input
  Sum4 : Sum  Inputs=+-  InputSameDT=on  SaturateOnIntegerOverflow=on  OutDataTypeStr=Inherit: Same as first input
  Unit Delay2 : UnitDelay  SampleTime=Ts  HasFrameUpgradeWarning=on
  Unit Delay5 : UnitDelay  InitialCondition=Vc_Initial  SampleTime=Ts  HasFrameUpgradeWarning=on
  Unit Delay6 : UnitDelay  InitialCondition=Vc_Initial  SampleTime=Ts  HasFrameUpgradeWarning=on
  Voltage Measurement : spsVoltageMeasurementLib/Voltage Measurement  PhasorSimulation=off  OutputType=Complex  PSBequivalent=0
  1 : PMIOPort  Side=Left
  2 : PMIOPort  Port=2  Side=Left
  Vc : Outport  VectorParamsAs1DForOutWhenUnconnected=off
  wires:
  Demux/1 -> Scope/1, [Vin]
  [Vin] -> Controlled Voltage Source/1
  Current Measurement1/1 -> [Icap]
  Product3/1 -> Sum3/1
  Demux/2 -> Scope/2, [Vbl]
  [Imod] -> Mux1/1
  Sum3/1 -> Gain4/1
  Unit Delay5/1 -> Sum4/2
  Gain5/1 -> Sum4/1
  Mux1/1 -> Unit Delay2/1
  Uref/1 -> Gain1/1
  Sum4/1 -> Vc/1, Product4/2
  Current Measurement/1 -> [Imod]
  Unit Delay2/1 -> Product3/2
  Discrete-Time Integrator1/1 -> Unit Delay6/1
  Product4/1 -> Demux/1
  [Vbl] -> Controlled Voltage Source1/1
  [Icap] -> Mux1/2
  Gain4/1 -> Discrete-Time Integrator1/1
  Unit Delay6/1 -> Gain5/1, Unit Delay5/1
  Gain1/1 -> Product3/1, Product4/1
  Voltage Measurement/1 -> [Vsm]
  [Vsm] -> Scope/3
  connections:
  Diode1/LConn1 -- Current Measurement/RConn1 -- Diode/RConn1
  Controlled Voltage Source1/LConn1 -- Diode/LConn1 -- 2/RConn1 -- Voltage Measurement/LConn2
  Controlled Voltage Source1/RConn1 -- Current Measurement1/RConn1
  Diode1/RConn1 -- Current Measurement1/LConn1
  Controlled Voltage Source/RConn1 -- 1/RConn1 -- Voltage Measurement/LConn1
  Controlled Voltage Source/LConn1 -- Current Measurement/LConn1

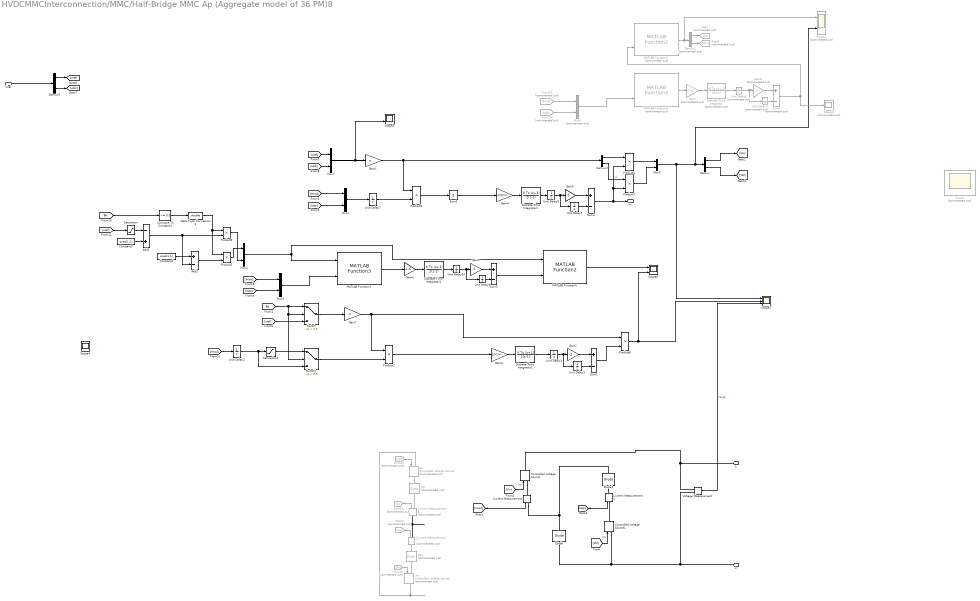
== system HVDCMMCInterconnection/MMC/Half-Bridge MMC Ap (Aggregate model of 36 PM)8 ==
  Uref : Inport
  Add1 : Sum  Inputs=+-
  Add2 : Sum  Inputs=-+
  Compare To Constant1 : simulink/Logic and Bit Operations/Compare To Constant  relop=<=  const=0.5  OutDataTypeStr=boolean
  Constant3 : Constant  Value=ones(1,1)
  Constant4 : Constant  Value=ones(1,1)
  Controlled Voltage Source : spsControlledVoltageSourceLib/Controlled Voltage Source  Initialize=on  Source_Type=AC  Amplitude=0  Phase=0  Frequency=0  Measurements=None
  Controlled Voltage Source1 : spsControlledVoltageSourceLib/Controlled Voltage Source  Initialize=on  Source_Type=AC  Amplitude=0  Phase=0  Frequency=0  Measurements=None
  Current Measurement : spsCurrentMeasurementLib/Current Measurement  PhasorSimulation=off  OutputType=Complex  PSBequivalent=0
  Current Measurement1 : spsCurrentMeasurementLib/Current Measurement  PhasorSimulation=off  OutputType=Complex  PSBequivalent=0
  Current Measurement7 : spsCurrentMeasurementLib/Current Measurement  Commented=on  PhasorSimulation=off  OutputType=Complex  PSBequivalent=0
  Current Measurement8 : spsCurrentMeasurementLib/Current Measurement  Commented=on  PhasorSimulation=off  OutputType=Complex  PSBequivalent=0
  Data Type Conversion2 : DataTypeConversion  OutDataTypeStr=double  SaturateOnIntegerOverflow=off  RndMeth=Floor
  Demux : Demux  Outputs=2
  Demux1 : Demux  Commented=on  Outputs=2
  Demux2 : Demux  Outputs=2
  Demux5 : Demux  Outputs=2
  Diode : spsDiodeLib/Diode  Ron=0.0001  Lon=0  Vf=0.0001  IC=0  UseSnubber=0  Rs=1e9  Cs=Cs_Diode  Measurements=off
  Diode1 : spsDiodeLib/Diode  Ron=0.0001  Lon=0  Vf=0.0001  IC=0  UseSnubber=0  Rs=1e9  Cs=Cs_Diode  Measurements=off
  Discrete-Time Integrator : DiscreteIntegrator  Commented=on  IntegratorMethod=Integration: Trapezoidal  gainval=1  InitialCondition=Vc_Initial  SampleTime=Ts  UpperSaturationLimit=5000  LowerSaturationLimit=500  ICPrevOutput=DiscIntNeverNeededParam  ICPrevScaledInput=DiscIntNeverNeededParam
  Discrete-Time Integrator1 : DiscreteIntegrator  IntegratorMethod=Integration: Trapezoidal  gainval=1  InitialCondition=Vc_Initial  SampleTime=Ts  UpperSaturationLimit=5000  LowerSaturationLimit=500  ICPrevOutput=DiscIntNeverNeededParam  ICPrevScaledInput=DiscIntNeverNeededParam
  Discrete-Time Integrator2 : DiscreteIntegrator  IntegratorMethod=Integration: Trapezoidal  gainval=1  InitialCondition=Vc_Initial  SampleTime=Ts  UpperSaturationLimit=5000  LowerSaturationLimit=500  ICPrevOutput=DiscIntNeverNeededParam  ICPrevScaledInput=DiscIntNeverNeededParam
  Discrete-Time Integrator3 : DiscreteIntegrator  IntegratorMethod=Integration: Trapezoidal  gainval=1  InitialCondition=Vc_Initial  SampleTime=Ts  UpperSaturationLimit=5000  LowerSaturationLimit=500  ICPrevOutput=DiscIntNeverNeededParam  ICPrevScaledInput=DiscIntNeverNeededParam
  Dp : spsDiodeLib/Diode  Commented=on  Ron=Ron_Diode  Lon=0  Vf=Vf_Diode  IC=0  UseSnubber=off  Rs=Rs_Diode  Cs=Cs_Diode  Measurements=off
  Dp1 : spsDiodeLib/Diode  Commented=on  Ron=Ron_Diode  Lon=0  Vf=Vf_Diode  IC=0  UseSnubber=off  Rs=Rs_Diode  Cs=Cs_Diode  Measurements=off
  From10 : From  Commented=on  GotoTag=Imod
  From14 : From  Commented=on  GotoTag=Icap
  From15 : From  Commented=on  GotoTag=Vp
  From16 : From  Commented=on  GotoTag=Vm
  Gain : Gain  Commented=on  Gain=-1./C
  Gain1 : Gain  Gain=n
  Gain2 : Gain  Gain=2
  Gain3 : Gain  Gain=1/(C*n)
  Gain4 : Gain  Gain=1/(C*n)
  Gain5 : Gain  Gain=2
  Gain6 : Gain  Gain=-1./C
  Gain7 : Gain  Gain=n
  Gain8 : Gain  Commented=on  Gain=2
  Gain9 : Gain  Gain=2
  Goto : Goto  Commented=on  GotoTag=Vp
  Goto18 : Goto  Commented=on  GotoTag=Ip
  Goto5 : Goto  Commented=on  GotoTag=Vm
  Goto8 : Goto  Commented=on  GotoTag=Im
  MATLAB Function1 : spsHalfBridgeMMCmodel/AVG Discrete/MATLAB Function3  n=1  ModelType=3
  MATLAB Function2 : spsHalfBridgeMMCmodel/AVG Discrete/MATLAB Function2  Commented=on  n=1  ModelType=3
  MATLAB Function3 : spsHalfBridgeMMCmodel/AVG Discrete/MATLAB Function3  Commented=on  n=1  ModelType=3
  MATLAB Function4 : spsHalfBridgeMMCmodel/AVG Discrete/MATLAB Function2  n=1  ModelType=3
  Mux{1..3,5,7} (5 alike) : Mux  Inputs=2
  Mux4 : Mux  Commented=on  Inputs=2
  Product{1..5,7..8} (7 alike) : Product
  Saturation : Saturate  UpperLimit=1  LowerLimit=-1
  Saturation2 : Saturate  UpperLimit=inf  LowerLimit=0
  Scope : Scope  Commented=on  NumInputPorts=2
  Scope1 : Scope  NumInputPorts=3
  Scope2 : Scope  Commented=on
  Scope3 : Scope  Commented=on  NumInputPorts=2
  Scope4 : Scope  NumInputPorts=2
  Scope5 : Scope  NumInputPorts=2
  Scope6 : Scope  NumInputPorts=2
  Sum1 : Sum  Inputs=+-  InputSameDT=on  SaturateOnIntegerOverflow=on  OutDataTypeStr=Inherit: Same as first input
  Sum2 : Sum  Commented=on  Inputs=+-  InputSameDT=on  SaturateOnIntegerOverflow=on  OutDataTypeStr=Inherit: Same as first input
  Sum3 : Sum  Inputs=1  InputSameDT=on  SaturateOnIntegerOverflow=on  OutDataTypeStr=Inherit: Same as first input
  Sum4 : Sum  Inputs=+-  InputSameDT=on  SaturateOnIntegerOverflow=on  OutDataTypeStr=Inherit: Same as first input
  Sum5 : Sum  Inputs=+-  InputSameDT=on  SaturateOnIntegerOverflow=on  OutDataTypeStr=Inherit: Same as first input
  Switch : Switch  Criteria=u2 > Threshold  Threshold=0.5  SaturateOnIntegerOverflow=off  InputSameDT=off
  Switch1 : Switch  Criteria=u2 > Threshold  Threshold=0.5  SaturateOnIntegerOverflow=off  InputSameDT=off
  Unit Delay{1,3,5..6,9..10} (6 alike) : UnitDelay  InitialCondition=Vc_Initial  SampleTime=Ts  HasFrameUpgradeWarning=on
  Unit Delay2 : UnitDelay  SampleTime=Ts  HasFrameUpgradeWarning=on
  Unit Delay4 : UnitDelay  Commented=on  InitialCondition=Vc_Initial  SampleTime=Ts  HasFrameUpgradeWarning=on
  Unit Delay7 : UnitDelay  SampleTime=Ts  HasFrameUpgradeWarning=on
  Unit Delay8 : UnitDelay  Commented=on  InitialCondition=Vc_Initial  SampleTime=Ts  HasFrameUpgradeWarning=on
  Vm : spsControlledVoltageSourceLib/Controlled Voltage Source  Commented=on  Initialize=off  Source_Type=AC  Amplitude=0  Phase=0  Frequency=0  Measurements=None
  Voltage Measurement : spsVoltageMeasurementLib/Voltage Measurement  PhasorSimulation=off  OutputType=Complex  PSBequivalent=0
  Vp : spsControlledVoltageSourceLib/Controlled Voltage Source  Commented=on  Initialize=off  Source_Type=AC  Amplitude=0  Phase=0  Frequency=0  Measurements=None
  1 : PMIOPort  Side=Left
  2 : PMIOPort  Port=2  Side=Left
  Vc : Outport  VectorParamsAs1DForOutWhenUnconnected=off
  wires:
  Demux/1 -> [Vin]
  [Vin] -> Controlled Voltage Source/1  "Vin"
  Product3/1 -> Sum3/1
  Demux/2 -> [Vbl]
  [Imod] -> Mux1/1
  Unit Delay5/1 -> Sum4/2
  Gain5/1 -> Sum4/1
  Sum4/1 -> Product7/2, Product4/2, Vc/1  "Vc"
  Discrete-Time Integrator1/1 -> Unit Delay6/1
  Mux2/1 -> Scope1/1, Scope3/2, Demux/1
  [Vbl] -> Controlled Voltage Source1/1  "Vbl"
  [Icap] -> Mux1/2
  Gain4/1 -> Discrete-Time Integrator1/1
  Unit Delay6/1 -> Gain5/1, Unit Delay5/1
  Mux1/1 -> Unit Delay7/1
  Mux7/1 -> Scope5/2, Gain1/1
  Gain3/1 -> Discrete-Time Integrator2/1
  Demux2/1 -> Product4/1
  Demux2/2 -> Product7/1
  Product4/1 -> Mux2/1
  Product7/1 -> Mux2/2
  Unit Delay3/1 -> Gain2/1, Unit Delay1/1
  Unit Delay1/1 -> Sum1/2
  Gain2/1 -> Sum1/1
  Discrete-Time Integrator2/1 -> Unit Delay3/1
  Product2/1 -> Gain3/1
  Sum1/1 -> Product8/2
  Demux5/2 -> [ublk]
  [uref] -> Mux7/1
  [ublk] -> Mux7/2
  Current Measurement/1 -> [Imod]
  Current Measurement1/1 -> [Icap]
  Unit Delay7/1 -> Product3/2
  [uref] -> Switch/3
  [Imod] -> Unit Delay2/1
  Saturation2/1 -> Switch1/1
  [Blk] -> Switch1/2, Switch/2, Switch/1
  Switch1/1 -> Product2/2
  Product8/1 -> Scope6/2, Scope1/2
  Unit Delay2/1 -> Saturation2/1, Switch1/3
  Gain1/1 -> Demux2/1, Product3/1
  Gain7/1 -> Product2/1, Product8/1
  Demux5/1 -> [uref]
  Uref/1 -> Demux5/1
  Voltage Measurement/1 -> Scope1/3  "Target"
  Gain8/1 -> Sum2/1
  Data Type Conversion2/1 -> Product5/1, Product1/1
  [Blk] -> Compare To Constant1/1
  Unit Delay4/1 -> Sum2/2
  Unit Delay8/1 -> Unit Delay4/1, Gain8/1
  Gain/1 -> Discrete-Time Integrator/1
  MATLAB Function2/1 -> Scope3/1, Demux1/1
  Add2/1 -> Add1/2, Product5/2
  MATLAB Function3/1 -> Gain/1
  Constant4/1 -> Add1/1
  Demux1/1 -> Goto/1
  [uref] -> Saturation/1
  Compare To Constant1/1 -> Data Type Conversion2/1
  Sum2/1 -> MATLAB Function2/2, Scope2/1
  Discrete-Time Integrator/1 -> Unit Delay8/1
  Demux1/2 -> Goto5/1
  Add1/1 -> Product1/2
  Product1/1 -> Mux3/1
  Constant3/1 -> Add2/2
  Saturation/1 -> Add2/1
  Sum3/1 -> Gain4/1
  From14/1 -> Mux4/2
  From10/1 -> Mux4/1
  Mux4/1 -> MATLAB Function3/2
  Product5/1 -> Mux3/2
  Switch/1 -> Gain7/1
  Mux5/1 -> MATLAB Function1/2
  [Imod] -> Mux5/1
  [Icap] -> Mux5/2
  Mux3/1 -> MATLAB Function1/1, MATLAB Function4/1
  Discrete-Time Integrator3/1 -> Unit Delay10/1
  Gain6/1 -> Discrete-Time Integrator3/1
  MATLAB Function1/1 -> Gain6/1
  Gain9/1 -> Sum5/1
  Unit Delay9/1 -> Sum5/2
  Unit Delay10/1 -> Unit Delay9/1, Gain9/1
  Sum5/1 -> MATLAB Function4/2
  MATLAB Function4/1 -> Scope6/1
  Current Measurement8/1 -> Goto18/1
  From16/1 -> Vm/1
  From15/1 -> Vp/1
  Current Measurement7/1 -> Goto8/1
  connections:
  Current Measurement/RConn1 -- Diode1/LConn1 -- Diode/RConn1
  Diode/LConn1 -- Voltage Measurement/LConn2 -- 2/RConn1 -- Controlled Voltage Source1/LConn1
  Controlled Voltage Source1/RConn1 -- Current Measurement1/RConn1
  Diode1/RConn1 -- Current Measurement1/LConn1
  1/RConn1 -- Voltage Measurement/LConn1 -- Controlled Voltage Source/RConn1
  Controlled Voltage Source/LConn1 -- Current Measurement/LConn1
  Vm/RConn1 -- Vp/LConn1
  Current Measurement8/LConn1 -- Current Measurement7/RConn1
  Vp/RConn1 -- Dp/RConn1
  Dp1/LConn1 -- Vm/LConn1
  Dp1/RConn1 -- Current Measurement7/LConn1
  Current Measurement8/RConn1 -- Dp/LConn1

== system HVDCMMCInterconnection/MMC/Meas_An ==
  An_I : spsCurrentMeasurementLib/Current Measurement  PhasorSimulation=off  OutputType=Complex  PSBequivalent=0
  An_V : spsVoltageMeasurementLib/Voltage Measurement  PhasorSimulation=off  OutputType=Complex  PSBequivalent=0
  I1 : PMIOPort  Side=Left
  I2 : PMIOPort  Port=2  Side=Left
  O1 : PMIOPort  Port=3  Side=Right
  O2 : PMIOPort  Port=4  Side=Right
  tag scope: I_Am=global, V12_Am=global
  wires:
  An_V/1 -> [V12_Am]
  An_I/1 -> [I_Am]
  connections:
  An_V/LConn2 -- O2/RConn1 -- I2/RConn1
  An_I/LConn1 -- O1/RConn1
  An_V/LConn1 -- An_I/RConn1 -- I1/RConn1

== system HVDCMMCInterconnection/MMC/Meas_Ap ==
  Ap_I : spsCurrentMeasurementLib/Current Measurement  PhasorSimulation=off  OutputType=Complex  PSBequivalent=0
  Ap_V : spsVoltageMeasurementLib/Voltage Measurement  PhasorSimulation=off  OutputType=Complex  PSBequivalent=0
  I1 : PMIOPort  Side=Left
  I2 : PMIOPort  Port=2  Side=Left
  O1 : PMIOPort  Port=3  Side=Right
  O2 : PMIOPort  Port=4  Side=Right
  tag scope: I_Ap=global, V12_Ap=global
  wires:
  Ap_I/1 -> [I_Ap]
  Ap_V/1 -> [V12_Ap]
  connections:
  Ap_I/RConn1 -- Ap_V/LConn1 -- I1/RConn1
  Ap_I/LConn1 -- O1/RConn1
  I2/RConn1 -- Ap_V/LConn2 -- O2/RConn1

== system HVDCMMCInterconnection/MMC/Meas_Bn ==
  Bn_I : spsCurrentMeasurementLib/Current Measurement  PhasorSimulation=off  OutputType=Complex  PSBequivalent=0
  Bn_V : spsVoltageMeasurementLib/Voltage Measurement  PhasorSimulation=off  OutputType=Complex  PSBequivalent=0
  I1 : PMIOPort  Side=Left
  I2 : PMIOPort  Port=2  Side=Left
  O1 : PMIOPort  Port=3  Side=Right
  O2 : PMIOPort  Port=4  Side=Right
  tag scope: I_Bm=global, V12_Bm=global
  wires:
  Bn_I/1 -> [I_Bm]
  Bn_V/1 -> [V12_Bm]
  connections:
  I1/RConn1 -- Bn_I/RConn1 -- Bn_V/LConn1
  Bn_I/LConn1 -- O1/RConn1
  I2/RConn1 -- O2/RConn1 -- Bn_V/LConn2

== system HVDCMMCInterconnection/MMC/Meas_Bp ==
  Bp_I : spsCurrentMeasurementLib/Current Measurement  PhasorSimulation=off  OutputType=Complex  PSBequivalent=0
  Bp_V : spsVoltageMeasurementLib/Voltage Measurement  PhasorSimulation=off  OutputType=Complex  PSBequivalent=0
  I1 : PMIOPort  Side=Left
  I2 : PMIOPort  Port=2  Side=Left
  O1 : PMIOPort  Port=3  Side=Right
  O2 : PMIOPort  Port=4  Side=Right
  tag scope: I_Bp=global, V12_Bp=global
  wires:
  Bp_V/1 -> [V12_Bp]
  Bp_I/1 -> [I_Bp]
  connections:
  Bp_V/LConn2 -- O2/RConn1 -- I2/RConn1
  Bp_I/LConn1 -- O1/RConn1
  Bp_V/LConn1 -- Bp_I/RConn1 -- I1/RConn1
